simulink model "simulate_data"  (R2016a)
settings: Solver=ode4  StartTime=0.0  StopTime=1  FixedStep=0.01  RelTol=1e-3
libraries: simulink x14
settings Model: Creator=callen  LastModifiedBy=callen
settings SolverCC: AutoInsertRateTranBlk=on
settings GRTTargetCC: GeneratePreprocessorConditionals=Use local settings

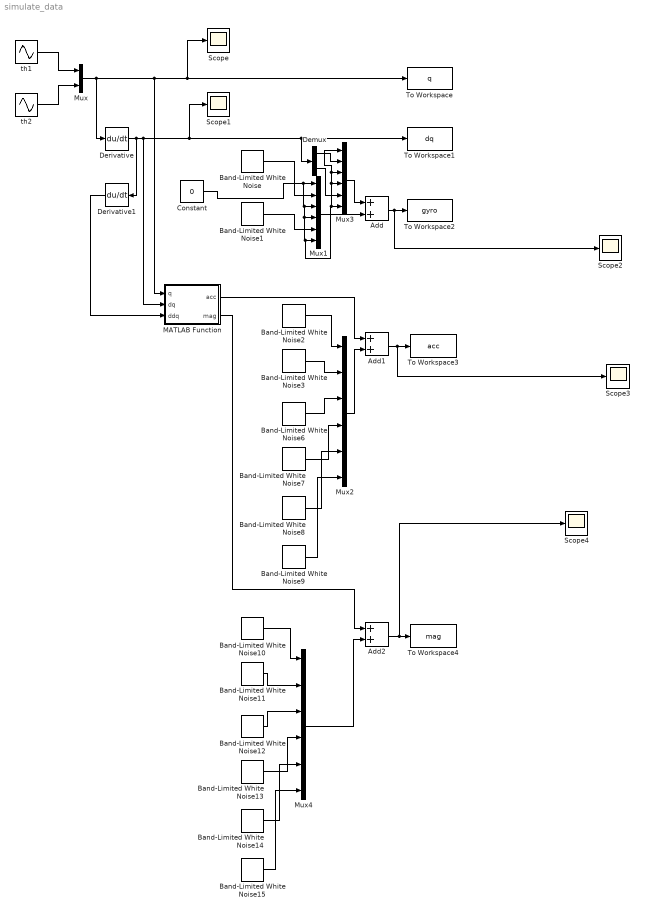
== system simulate_data ==
  Add : Sum
  Add1 : Sum
  Add2 : Sum
  Band-Limited White Noise{,1..3,6..15} (14 alike) : simulink/Sources/Band-Limited White Noise  Cov=0.01  Ts=0.1  seed=[23341]
  Constant : Constant  Value=0
  Demux : Demux  Outputs=2
  Derivative : Derivative
  Derivative1 : Derivative
  MATLAB Function : MATLAB Function  TreatAsAtomicUnit=on
  Mux : Mux  Inputs=2
  Mux{1..4} (4 alike) : Mux  Inputs=6
  Scope{,1..4} (5 alike) : Scope
  To Workspace : ToWorkspace  VariableName=q  SaveFormat=Structure With Time  SampleTime=0.01
  To Workspace1 : ToWorkspace  VariableName=dq  SaveFormat=Structure With Time  SampleTime=0.01
  To Workspace2 : ToWorkspace  VariableName=gyro  SaveFormat=Structure With Time  SampleTime=0.01
  To Workspace3 : ToWorkspace  VariableName=acc  SaveFormat=Structure With Time  SampleTime=0.01
  To Workspace4 : ToWorkspace  VariableName=mag  SaveFormat=Structure With Time  SampleTime=0.01
  th1 : Sin  Amplitude=pi/2  SampleTime=0
  th2 : Sin  Amplitude=pi/2  SampleTime=0
  wires:
  th1/1 -> Mux/1
  th2/1 -> Mux/2
  Derivative/1 -> Derivative1/1, Demux/1, To Workspace1/1, Scope1/1, MATLAB Function/2(dq)
  Mux/1 -> Scope/1, To Workspace/1, MATLAB Function/1(q), Derivative/1
  Mux1/1 -> Add/2
  Add/1 -> Scope2/1, To Workspace2/1
  MATLAB Function/1(acc) -> Add1/1
  Band-Limited White Noise2/1 -> Mux2/1
  Band-Limited White Noise3/1 -> Mux2/2
  Mux2/1 -> Add1/2
  Add1/1 -> Scope3/1, To Workspace3/1
  MATLAB Function/2(mag) -> Add2/1
  Mux4/1 -> Add2/2
  Add2/1 -> Scope4/1, To Workspace4/1
  Derivative1/1 -> MATLAB Function/3(ddq)
  Band-Limited White Noise6/1 -> Mux2/3
  Band-Limited White Noise7/1 -> Mux2/4
  Band-Limited White Noise8/1 -> Mux2/5
  Band-Limited White Noise9/1 -> Mux2/6
  Band-Limited White Noise10/1 -> Mux4/1
  Band-Limited White Noise11/1 -> Mux4/2
  Band-Limited White Noise12/1 -> Mux4/3
  Band-Limited White Noise13/1 -> Mux4/4
  Band-Limited White Noise14/1 -> Mux4/5
  Band-Limited White Noise15/1 -> Mux4/6
  Band-Limited White Noise/1 -> Mux1/2
  Band-Limited White Noise1/1 -> Mux1/5
  Constant/1 -> Mux3/1, Mux3/3, Mux3/4, Mux3/6, Mux1/6, Mux1/4, Mux1/3, Mux1/1
  Mux3/1 -> Add/1
  Demux/1 -> Mux3/2
  Demux/2 -> Mux3/5

== matlab function simulate_data/MATLAB Function ==
  data: q input; acc output; dq input; mag output; ddq input
function [acc,mag]= fcn(q,dq,ddq)
%#codegen

th1=q(1);
th2=q(2);

dth1=dq(1);
dth2=dq(2);

ddth1=ddq(1);
ddth2=ddq(2);

l1=1;
l2=1;
g=9.81;
mag_vec=[0.7071;0;0.7071];


beam1_acc=[- l1*cos(th1)*dth1^2 - ddth1*l1*sin(th1);...
    0;...
    l1*sin(th1)*dth1^2 - ddth1*l1*cos(th1)];  
beam2_acc=[- l1*cos(th1)*dth1^2 - l2*cos(th2)*dth2^2 - ddth1*l1*sin(th1) - ddth2*l2*sin(th2);...
    0;...
    l1*sin(th1)*dth1^2 + l2*sin(th2)*dth2^2 - ddth1*l1*cos(th1) - ddth2*l2*cos(th2)];

acc1=R(th1).'*[0;0;g]+R(th1).'*beam1_acc;
acc2=R(th2).'*[0;0;g]+R(th2).'*beam2_acc;

mag1=R(th1).'*mag_vec;
mag2=R(th2).'*mag_vec;

acc=[acc1;acc2];
mag=[mag1;mag2];
